simulink model "CircuitForLoad_SimuLink"  (R2022b)
settings: Solver=VariableStepAuto  StartTime=0.0  StopTime=5.0  RelTol=1e-3
libraries: ee_lib x7, fl_lib x6, nesl_utility x4
settings Model: Creator=monster  LastModifiedBy=monster

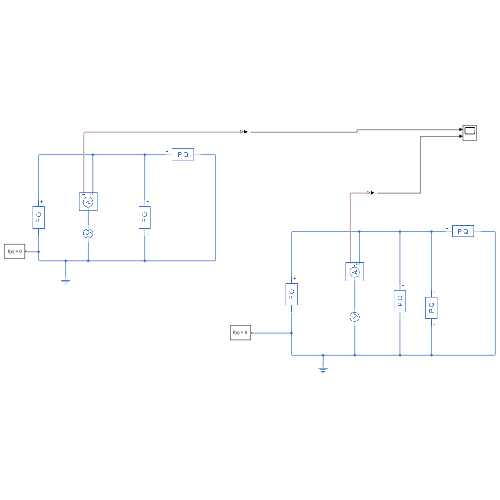
[thumbnail: Simulink's stored preview of the top-level diagram]
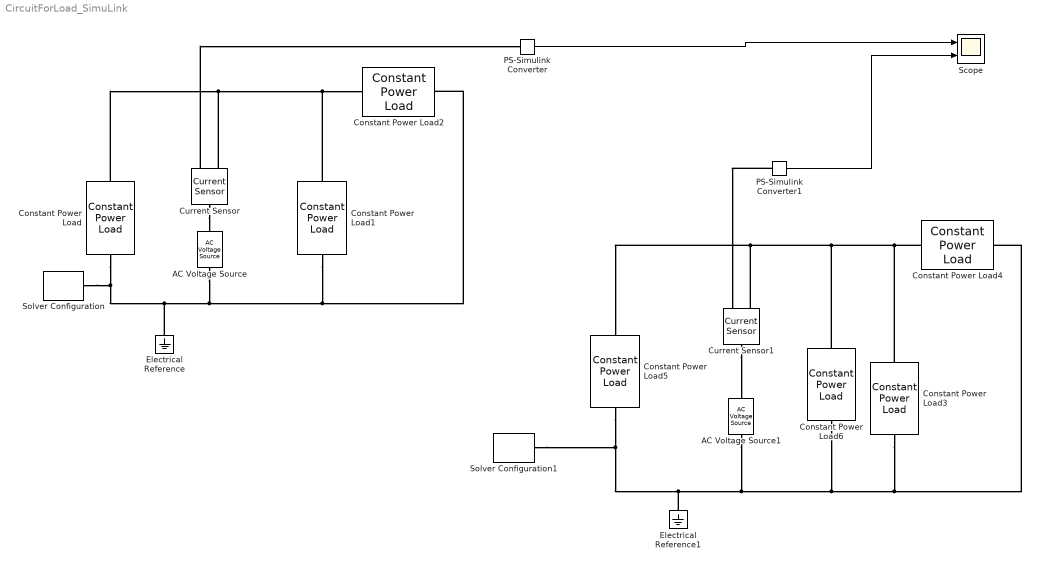
== system CircuitForLoad_SimuLink ==
  AC Voltage Source : fl_lib/Electrical/Electrical Sources/AC Voltage Source  amp=325 V  shift=0 deg  frequency=50 Hz  omega=0 rad/s
  AC Voltage Source1 : fl_lib/Electrical/Electrical Sources/AC Voltage Source  amp=325 V  shift=0 deg  frequency=50 Hz  omega=0 rad/s
  Constant Power Load : ee_lib/Passive/Constant Power Load  load_type=ee.enum.dc_ac.ac  consumed_power=100 W  min_supply_voltage=20 V  G_reverse=1e-6 S  deltaV=1e-3 V  active_power=10000 W  reactive_power=10000 A*V  f0=50 Hz  Vrms_min=230 V  enable_fault=simscape.enum.onoff.off  fault_action=simscape.enum.assert.action.none  t_fault=1 s  open_conductance=1e-4 S
      settings: InternalSimscapePortConfiguration="{\"Bottom\":[],\"Left\":[{\"id\":\"p\",\"label\":\"+\",\"type\":\"foundation.electrical.electrical\"}],\"Right\":[{\"id\":\"n\",\"label\":\"-\",\"type\":\"foundation.electrical.electrical\"}],\"Top\":[]}"
  Constant Power Load1 : ee_lib/Passive/Constant Power Load  load_type=ee.enum.dc_ac.ac  consumed_power=100 W  min_supply_voltage=20 V  G_reverse=1e-6 S  deltaV=1e-3 V  active_power=5000 W  reactive_power=6097.5 A*V  f0=50 Hz  Vrms_min=230 V  enable_fault=simscape.enum.onoff.off  fault_action=simscape.enum.assert.action.none  t_fault=1 s  open_conductance=1e-4 S
      settings: InternalSimscapePortConfiguration="{\"Bottom\":[],\"Left\":[{\"id\":\"p\",\"label\":\"+\",\"type\":\"foundation.electrical.electrical\"}],\"Right\":[{\"id\":\"n\",\"label\":\"-\",\"type\":\"foundation.electrical.electrical\"}],\"Top\":[]}"
  Constant Power Load2 : ee_lib/Passive/Constant Power Load  load_type=ee.enum.dc_ac.ac  consumed_power=100 W  min_supply_voltage=20 V  G_reverse=1e-6 S  deltaV=1e-3 V  active_power=18090 W  reactive_power=27000 A*V  f0=50 Hz  Vrms_min=230 V  enable_fault=simscape.enum.onoff.off  fault_action=simscape.enum.assert.action.none  t_fault=1 s  open_conductance=1e-4 S
      settings: InternalSimscapePortConfiguration="{\"Bottom\":[],\"Left\":[{\"id\":\"p\",\"label\":\"+\",\"type\":\"foundation.electrical.electrical\"}],\"Right\":[{\"id\":\"n\",\"label\":\"-\",\"type\":\"foundation.electrical.electrical\"}],\"Top\":[]}"
  Constant Power Load3 : ee_lib/Passive/Constant Power Load  load_type=ee.enum.dc_ac.ac  consumed_power=100 W  min_supply_voltage=20 V  G_reverse=1e-6 S  deltaV=1e-3 V  active_power=0.000000000001 W  reactive_power=5677 A*V  f0=50 Hz  Vrms_min=230 V  enable_fault=simscape.enum.onoff.off  fault_action=simscape.enum.assert.action.none  t_fault=1 s  open_conductance=1e-4 S
      settings: InternalSimscapePortConfiguration="{\"Bottom\":[],\"Left\":[{\"id\":\"p\",\"label\":\"+\",\"type\":\"foundation.electrical.electrical\"}],\"Right\":[{\"id\":\"n\",\"label\":\"-\",\"type\":\"foundation.electrical.electrical\"}],\"Top\":[]}"
  Constant Power Load4 : ee_lib/Passive/Constant Power Load  load_type=ee.enum.dc_ac.ac  consumed_power=100 W  min_supply_voltage=20 V  G_reverse=1e-6 S  deltaV=1e-3 V  active_power=18090 W  reactive_power=27000 A*V  f0=50 Hz  Vrms_min=230 V  enable_fault=simscape.enum.onoff.off  fault_action=simscape.enum.assert.action.none  t_fault=1 s  open_conductance=1e-4 S
      settings: InternalSimscapePortConfiguration="{\"Bottom\":[],\"Left\":[{\"id\":\"p\",\"label\":\"+\",\"type\":\"foundation.electrical.electrical\"}],\"Right\":[{\"id\":\"n\",\"label\":\"-\",\"type\":\"foundation.electrical.electrical\"}],\"Top\":[]}"
  Constant Power Load5 : ee_lib/Passive/Constant Power Load  load_type=ee.enum.dc_ac.ac  consumed_power=100 W  min_supply_voltage=20 V  G_reverse=1e-6 S  deltaV=1e-3 V  active_power=10000 W  reactive_power=10000 A*V  f0=50 Hz  Vrms_min=230 V  enable_fault=simscape.enum.onoff.off  fault_action=simscape.enum.assert.action.none  t_fault=1 s  open_conductance=1e-4 S
      settings: InternalSimscapePortConfiguration="{\"Bottom\":[],\"Left\":[{\"id\":\"p\",\"label\":\"+\",\"type\":\"foundation.electrical.electrical\"}],\"Right\":[{\"id\":\"n\",\"label\":\"-\",\"type\":\"foundation.electrical.electrical\"}],\"Top\":[]}"
  Constant Power Load6 : ee_lib/Passive/Constant Power Load  load_type=ee.enum.dc_ac.ac  consumed_power=100 W  min_supply_voltage=20 V  G_reverse=1e-6 S  deltaV=1e-3 V  active_power=5000 W  reactive_power=6097.5 A*V  f0=50 Hz  Vrms_min=230 V  enable_fault=simscape.enum.onoff.off  fault_action=simscape.enum.assert.action.none  t_fault=1 s  open_conductance=1e-4 S
      settings: InternalSimscapePortConfiguration="{\"Bottom\":[],\"Left\":[{\"id\":\"p\",\"label\":\"+\",\"type\":\"foundation.electrical.electrical\"}],\"Right\":[{\"id\":\"n\",\"label\":\"-\",\"type\":\"foundation.electrical.electrical\"}],\"Top\":[]}"
  Current Sensor : fl_lib/Electrical/Electrical Sensors/Current Sensor
  Current Sensor1 : fl_lib/Electrical/Electrical Sensors/Current Sensor
  Electrical Reference : fl_lib/Electrical/Electrical Elements/Electrical Reference
  Electrical Reference1 : fl_lib/Electrical/Electrical Elements/Electrical Reference
  PS-Simulink Converter : nesl_utility/PS-Simulink Converter  PhysicalDomain=network_engine_domain  SubClassName=ps_output  LeftPortType=input  RightPortType=output  PseudoPeriodic=off  Frequencies=[]  VectorFormat=inherit  Unit=inherit  AffineConversion=off
  PS-Simulink Converter1 : nesl_utility/PS-Simulink Converter  PhysicalDomain=network_engine_domain  SubClassName=ps_output  LeftPortType=input  RightPortType=output  PseudoPeriodic=off  Frequencies=[]  VectorFormat=inherit  Unit=inherit  AffineConversion=off
  Scope : Scope  NumInputPorts=2
  Solver Configuration : nesl_utility/Solver Configuration  PhysicalDomain=network_engine_domain  SubClassName=solver  LeftPortType=input  RightPortType=generic  Tones=[]  Harmonics=[]  SimulateNoise=off  Profile=off  UseLocalSampling=off  EnableSwitchedLinearOptims=on  FrequencyDomain=off  UseCCode=off  RelTol=0.001  AbsTol=0.001  MinStep=1e-09  ToWorkspace=off  RevertToSquareIcSolve=off  NumHomotopyIterations=100  PhasorMode=off  PhasorModeNumHarmonics=1  ConsistencySolver=NEWTON_XTOL_AFTER_FTOL  IndexReductionMethod=DerivativeReplacement  DoDC=off  ResidualTolerance=1e-09  ConsistencyTolSource=GLOBAL  ConsistencyAbsTol=0.001  ConsistencyRelTol=0.001  ConsistencyTolFactor=0.001  UseLocalSolver=off  LocalSolverChoice=NE_BACKWARD_EULER_ADVANCER  ResolveIndetEquations=on  FunctionEvalNumThread=1  LocalSolverSampleTime=0.001  DoFixedCost=off  MaxNonlinIter=3  MaxModeIter=2  ComputeImpulses=off  ImpulseIterations=2  LinearAlgebra=auto  LinearAlgebraNumThread=0  EquationFormulation=NE_TIME_EF  DelaysMemoryBudget=1024  AutomaticFiltering=on  FilteringTimeConstant=0.001  PartitionStorageMethod=AS_NEEDED  PartitionMemoryBudget=1024  PartitionMethod=ROBUST
  Solver Configuration1 : nesl_utility/Solver Configuration  PhysicalDomain=network_engine_domain  SubClassName=solver  LeftPortType=input  RightPortType=generic  Tones=[]  Harmonics=[]  SimulateNoise=off  Profile=off  UseLocalSampling=off  EnableSwitchedLinearOptims=on  FrequencyDomain=off  UseCCode=off  RelTol=0.001  AbsTol=0.001  MinStep=1e-09  ToWorkspace=off  RevertToSquareIcSolve=off  NumHomotopyIterations=100  PhasorMode=off  PhasorModeNumHarmonics=1  ConsistencySolver=NEWTON_XTOL_AFTER_FTOL  IndexReductionMethod=DerivativeReplacement  DoDC=off  ResidualTolerance=1e-09  ConsistencyTolSource=GLOBAL  ConsistencyAbsTol=0.001  ConsistencyRelTol=0.001  ConsistencyTolFactor=0.001  UseLocalSolver=off  LocalSolverChoice=NE_BACKWARD_EULER_ADVANCER  ResolveIndetEquations=on  FunctionEvalNumThread=1  LocalSolverSampleTime=0.001  DoFixedCost=off  MaxNonlinIter=3  MaxModeIter=2  ComputeImpulses=off  ImpulseIterations=2  LinearAlgebra=auto  LinearAlgebraNumThread=0  EquationFormulation=NE_TIME_EF  DelaysMemoryBudget=1024  AutomaticFiltering=on  FilteringTimeConstant=0.001  PartitionStorageMethod=AS_NEEDED  PartitionMemoryBudget=1024  PartitionMethod=ROBUST
  wires:
  PS-Simulink Converter/1 -> Scope/1
  PS-Simulink Converter1/1 -> Scope/2
  connections:
  Constant Power Load/RConn1 -- Solver Configuration/RConn1 -- Electrical Reference/LConn1 -- AC Voltage Source/RConn1 -- Constant Power Load1/RConn1 -- Constant Power Load2/RConn1
  Current Sensor/RConn2 -- Constant Power Load/LConn1 -- Constant Power Load1/LConn1 -- Constant Power Load2/LConn1
  Current Sensor/LConn1 -- AC Voltage Source/LConn1
  Current Sensor/RConn1 -- PS-Simulink Converter/LConn1
  Constant Power Load5/RConn1 -- Solver Configuration1/RConn1 -- Electrical Reference1/LConn1 -- AC Voltage Source1/RConn1 -- Constant Power Load6/RConn1 -- Constant Power Load3/RConn1 -- Constant Power Load4/RConn1
  Constant Power Load4/LConn1 -- Constant Power Load3/LConn1 -- Constant Power Load6/LConn1 -- Current Sensor1/RConn2 -- Constant Power Load5/LConn1
  Current Sensor1/LConn1 -- AC Voltage Source1/LConn1
  PS-Simulink Converter1/LConn1 -- Current Sensor1/RConn1
